simulink model "dram_acc_test8sim"  (Simulink 6.2)
settings: Solver=ode45  StartTime=0.0  StopTime=300000  RelTol=1e-3
undefined symbols (not defined in the file): ant_bits, blockCountBits, blockRowBits
libraries: xbsIndex_r3 x656, xps_library x19, casper_library x10
(part 4 of 4)

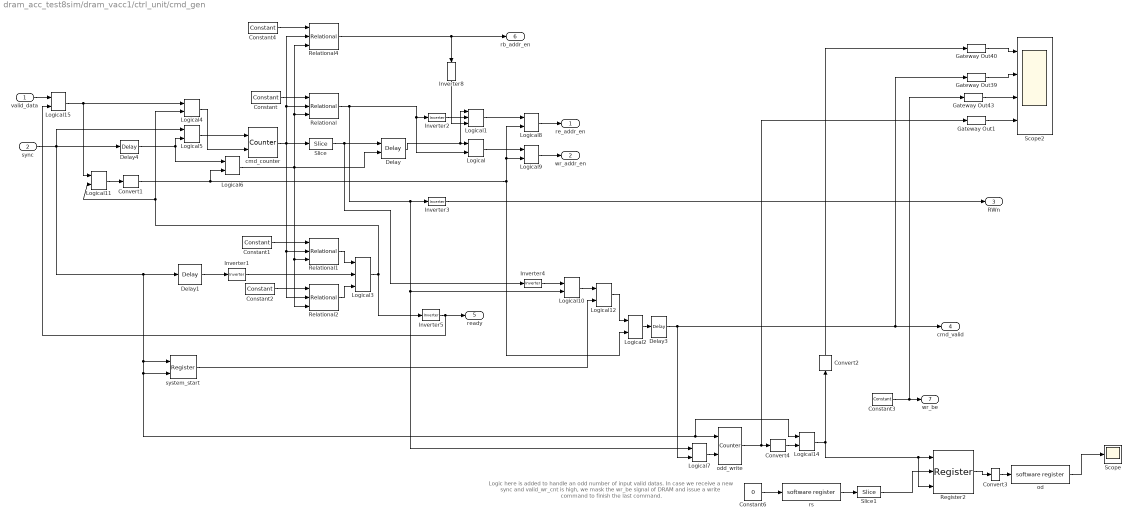
== system dram_acc_test8sim/dram_vacc1/ctrl_unit/cmd_gen ==
  note: Logic here is added to handle an  odd number of input valid datas.
      | In case we receive a new sync and valid_wr_cnt is high, we mask the wr_be
      | signal of DRAM and issue a write command to finish the last command.
  valid_data : Inport  Port=1  LatchInput=off
  sync : Inport  Port=2  LatchInput=off
  Constant : xbsIndex_r3/Constant  const=burst_length-1  equ=P=C  arith_type=Unsigned  n_bits=ceil(log2(2*burst_length+2))  bin_pt=0  opselect=C  inp2=PCIN>>17  opr=+  inp1=P  carry=CIN  iostate=0  explicit_period=on  period=1  dbl_ovrd=off
  Constant1 : xbsIndex_r3/Constant  const=burst_length-1  equ=P=C  arith_type=Unsigned  n_bits=ceil(log2(2*burst_length+2))  bin_pt=0  opselect=C  inp2=PCIN>>17  opr=+  inp1=P  carry=CIN  iostate=0  explicit_period=on  period=1  dbl_ovrd=off
  Constant2 : xbsIndex_r3/Constant  const=2*burst_length+2-1  equ=P=C  arith_type=Unsigned  n_bits=ceil(log2(2*burst_length+2))  bin_pt=0  opselect=C  inp2=PCIN>>17  opr=+  inp1=P  carry=CIN  iostate=0  explicit_period=on  period=1  dbl_ovrd=off
  Constant3 : xbsIndex_r3/Constant  const=2^18-1  equ=P=C  arith_type=Unsigned  n_bits=18  bin_pt=0  opselect=C  inp2=PCIN>>17  opr=+  inp1=P  carry=CIN  iostate=0  explicit_period=on  period=1  dbl_ovrd=off
  Constant4 : xbsIndex_r3/Constant  const=2*burst_length  equ=P=C  arith_type=Unsigned  n_bits=ceil(log2(2*burst_length+2))  bin_pt=0  opselect=C  inp2=PCIN>>17  opr=+  inp1=P  carry=CIN  iostate=0  explicit_period=on  period=1  dbl_ovrd=off
  Constant6 : Constant  Value=0
  Convert1 : xbsIndex_r3/Convert  arith_type=Boolean  n_bits=31  bin_pt=0  quantization=Truncate  overflow=Wrap  latency=0  explicit_period=on  period=1  dbl_ovrd=off  show_param=off  inserted_by_tool=off  pipeline=off
      settings: xl_area=[0, 0, 0, 0, 0, 0, 0]
  Convert2 : xbsIndex_r3/Convert  Orientation=up  arith_type=Boolean  n_bits=31  bin_pt=0  quantization=Truncate  overflow=Wrap  latency=1  explicit_period=on  period=1  dbl_ovrd=off  show_param=off  inserted_by_tool=off  pipeline=off
      settings: xl_area=[0, 0, 0, 0, 0, 0, 0]
  Convert3 : xbsIndex_r3/Convert  arith_type=Unsigned  n_bits=32  bin_pt=0  quantization=Truncate  overflow=Wrap  latency=0  explicit_period=on  period=1  dbl_ovrd=off  show_param=off  inserted_by_tool=off  pipeline=off
      settings: xl_area=[0, 0, 0, 0, 0, 0, 0]
  Convert4 : xbsIndex_r3/Convert  arith_type=Boolean  n_bits=31  bin_pt=0  quantization=Truncate  overflow=Wrap  latency=0  explicit_period=on  period=1  dbl_ovrd=off  show_param=off  inserted_by_tool=off  pipeline=off
      settings: xl_area=[0, 0, 0, 0, 0, 0, 0]
  Delay : xbsIndex_r3/Delay  latency=1  reg_retiming=off  explicit_period=off  period=1  en=on  accept_only_valid=off  init_zero=on  dbl_ovrd=off  show_param=off
      settings: xl_area=[0, 0, 0, 0, 0, 0, 0]
  Delay1 : xbsIndex_r3/Delay  latency=1  reg_retiming=off  explicit_period=off  period=1  en=off  accept_only_valid=off  init_zero=on  dbl_ovrd=off  show_param=off
      settings: xl_area=[0, 0, 0, 0, 0, 0, 0]
  Delay3 : xbsIndex_r3/Delay  latency=1  reg_retiming=off  explicit_period=on  period=1  en=off  accept_only_valid=off  init_zero=on  dbl_ovrd=off  show_param=off
      settings: xl_area=[0, 0, 0, 0, 0, 0, 0]
  Delay4 : xbsIndex_r3/Delay  latency=1  reg_retiming=off  explicit_period=on  period=1  en=off  accept_only_valid=off  init_zero=on  dbl_ovrd=off  show_param=off
      settings: xl_area=[0, 0, 0, 0, 0, 0, 0]
  Gateway Out{1,39..40,43} (4 alike) : xbsIndex_r3/Gateway Out  output_type=Double  nbits=8  bin_pt=6  arith_type=Boolean  quantization=Truncate  overflow=Wrap  hdl_port=off  timing_constraint=None  locs_specified=off  LOCs={}  needs_fixed_name=off  show_param=off
      settings: xl_area=[0, 0, 0, 0, 0, 0, 0]
  Inverter{1..5} (5 alike) : xbsIndex_r3/Inverter  latency=0  explicit_period=off  period=1  en=off  dbl_ovrd=off  show_param=off
      settings: xl_area=[0, 0, 0, 0, 0, 0, 0]
  Inverter8 : xbsIndex_r3/Inverter  Orientation=down  latency=0  explicit_period=off  period=1  en=off  dbl_ovrd=off  show_param=off
      settings: xl_area=[0, 0, 0, 0, 0, 0, 0]
  Logical{,2,7..9,12,14..15} (8 alike) : xbsIndex_r3/Logical  logical_function=AND  inputs=2  precision=Full  arith_type=Unsigned  n_bits=8  bin_pt=2  align_bp=on  latency=0  explicit_period=on  period=1  en=off  dbl_ovrd=off  show_param=off
      settings: xl_area=[0, 0, 0, 0, 0, 0, 0]
  Logical1 : xbsIndex_r3/Logical  logical_function=AND  inputs=3  precision=Full  arith_type=Unsigned  n_bits=8  bin_pt=2  align_bp=on  latency=0  explicit_period=on  period=1  en=off  dbl_ovrd=off  show_param=off
      settings: xl_area=[0, 0, 0, 0, 0, 0, 0]
  Logical10 : xbsIndex_r3/Logical  logical_function=OR  inputs=2  precision=Full  arith_type=Unsigned  n_bits=8  bin_pt=2  align_bp=on  latency=0  explicit_period=on  period=1  en=off  dbl_ovrd=off  show_param=off
      settings: xl_area=[0, 0, 0, 0, 0, 0, 0]
  Logical11 : xbsIndex_r3/Logical  logical_function=OR  inputs=2  precision=Full  arith_type=Unsigned  n_bits=8  bin_pt=2  align_bp=on  latency=0  explicit_period=on  period=1  en=off  dbl_ovrd=off  show_param=off
      settings: xl_area=[0, 0, 0, 0, 0, 0, 0]
  Logical3 : xbsIndex_r3/Logical  logical_function=AND  inputs=3  precision=Full  arith_type=Unsigned  n_bits=8  bin_pt=2  align_bp=on  latency=0  explicit_period=off  period=1  en=off  dbl_ovrd=off  show_param=off
      settings: xl_area=[0, 0, 0, 0, 0, 0, 0]
  Logical4 : xbsIndex_r3/Logical  logical_function=OR  inputs=2  precision=Full  arith_type=Unsigned  n_bits=8  bin_pt=2  align_bp=on  latency=0  explicit_period=off  period=1  en=off  dbl_ovrd=off  show_param=off
      settings: xl_area=[0, 0, 0, 0, 0, 0, 0]
  Logical5 : xbsIndex_r3/Logical  logical_function=OR  inputs=2  precision=Full  arith_type=Unsigned  n_bits=8  bin_pt=2  align_bp=on  latency=0  explicit_period=off  period=1  en=off  dbl_ovrd=off  show_param=off
      settings: xl_area=[0, 0, 0, 0, 0, 0, 0]
  Logical6 : xbsIndex_r3/Logical  logical_function=OR  inputs=2  precision=Full  arith_type=Unsigned  n_bits=8  bin_pt=2  align_bp=on  latency=0  explicit_period=on  period=1  en=off  dbl_ovrd=off  show_param=off
      settings: xl_area=[0, 0, 0, 0, 0, 0, 0]
  Register2 : xbsIndex_r3/Register  init=0  reg_only_valid=off  explicit_period=off  period=1  rst=on  en=on  out_en=off  dbl_ovrd=off  show_param=off
      settings: xl_area=[0, 0, 0, 0, 0, 0, 0]
  Relational : xbsIndex_r3/Relational  mode=a>=b  latency=1  explicit_period=on  period=1  en=on  dbl_ovrd=off  show_param=off
      settings: xl_area=[0, 0, 0, 0, 0, 0, 0]
  Relational1 : xbsIndex_r3/Relational  mode=a<=b  latency=1  explicit_period=on  period=1  en=on  dbl_ovrd=off  show_param=off
      settings: xl_area=[0, 0, 0, 0, 0, 0, 0]
  Relational2 : xbsIndex_r3/Relational  mode=a!=b  latency=1  explicit_period=off  period=1  en=on  dbl_ovrd=off  show_param=off
      settings: xl_area=[0, 0, 0, 0, 0, 0, 0]
  Relational4 : xbsIndex_r3/Relational  mode=a<=b  latency=1  explicit_period=on  period=1  en=on  dbl_ovrd=off  show_param=off
      settings: xl_area=[0, 0, 0, 0, 0, 0, 0]
  Scope : Scope
      settings: SaveName=ScopeData34
  Scope2 : Scope  NumInputPorts=4
      settings: YMin=-1~0~262143~0  YMax=1~1~262143~1  SaveName=ScopeData12
  Slice : xbsIndex_r3/Slice  mode=Lower Bit Location + Width  nbits=1  bit1=0  base1=MSB of Input  bit0=0  base0=LSB of Input  boolean_output=on  explicit_period=off  period=1  dbl_ovrd=off
  Slice1 : xbsIndex_r3/Slice  mode=Lower Bit Location + Width  nbits=1  bit1=0  base1=MSB of Input  bit0=0  base0=LSB of Input  boolean_output=on  explicit_period=off  period=1  dbl_ovrd=off
  cmd_counter : xbsIndex_r3/Counter  cnt_type=Count Limited  n_bits=ceil(log2(2*burst_length+2))  bin_pt=0  arith_type=Unsigned  start_count=0  cnt_to=2*burst_length+2-1  cnt_by_val=1  operation=Up  explicit_period=on  period=1  load_pin=off  rst=on  en=on  dbl_ovrd=off  show_param=off  use_rpm=on  gen_core=off
      settings: xl_area=[0, 0, 0, 0, 0, 0, 0]
  od : xps_library/software register  Tag=xps:sw_reg  io_dir=To Processor  arith_type=Unsigned  bitwidth=32  bin_pt=0  sample_period=1  gw_name=dram_acc_test8_dram_vacc1_ctrl_unit_cmd_gen_od_user_data_in
  odd_write : xbsIndex_r3/Counter  cnt_type=Free Running  n_bits=1  bin_pt=0  arith_type=Unsigned  start_count=0  cnt_to=2*burst_length+2-1  cnt_by_val=1  operation=Up  explicit_period=on  period=1  load_pin=off  rst=on  en=on  dbl_ovrd=off  show_param=off  use_rpm=on  gen_core=off
      settings: xl_area=[0, 0, 0, 0, 0, 0, 0]
  rs : xps_library/software register  Tag=xps:sw_reg  io_dir=From Processor  arith_type=Unsigned  bitwidth=32  bin_pt=0  sample_period=1  gw_name=dram_acc_test8_dram_vacc1_ctrl_unit_cmd_gen_rs_user_data_out
  system_start : xbsIndex_r3/Register  init=0  reg_only_valid=off  explicit_period=off  period=1  rst=off  en=on  out_en=off  dbl_ovrd=off  show_param=off
      settings: xl_area=[0, 0, 0, 0, 0, 0, 0]
  re_addr_en : Outport
  wr_addr_en : Outport  Port=2
  RWn : Outport  Port=3
  cmd_valid : Outport  Port=4
  ready : Outport  Port=5
  rb_addr_en : Outport  Port=6
  wr_be : Outport  Port=7
  wires:
  Logical9/1 -> wr_addr_en/1
  Logical8/1 -> re_addr_en/1
  Logical15/1 -> Logical4/1, Logical11/1
  Inverter8/1 -> Logical1/3
  Relational4/1 -> rb_addr_en/1, Inverter8/1
  Constant4/1 -> Relational4/1
  Logical6/1 -> Delay/2, Relational4/3, Relational/3, Relational1/3, Relational2/3
  Delay4/1 -> Logical6/1, Logical5/2
  Logical5/1 -> cmd_counter/1
  Logical2/1 -> Delay3/1
  Logical12/1 -> Logical2/1
  Convert1/1 -> Logical2/2, Logical8/2, Logical9/2, Logical6/2
  Inverter5/1 -> Logical15/2, ready/1
  Inverter4/1 -> Logical10/1
  Logical10/1 -> Logical12/1
  Inverter3/1 -> RWn/1
  Inverter2/1 -> Logical1/2
  system_start/1 -> Logical12/2
  Logical4/1 -> cmd_counter/2
  Logical3/1 -> Logical11/2, Logical4/2, Inverter5/1
  valid_data/1 -> Logical15/1
  Delay1/1 -> Inverter1/1
  Inverter1/1 -> Logical3/2
  Relational2/1 -> Logical3/3
  Constant2/1 -> Relational2/1
  Relational1/1 -> Logical3/1
  Constant1/1 -> Relational1/1
  Delay/1 -> Logical/1, Logical1/1
  Relational/1 -> Inverter3/1, Logical10/2, Logical7/1, Logical/2, Inverter2/1
  Slice/1 -> Inverter4/1, Delay/1
  Logical1/1 -> Logical8/1
  Logical/1 -> Logical9/1
  Logical11/1 -> Convert1/1
  Constant/1 -> Relational/1
  cmd_counter/1 -> Relational2/2, Relational1/2, Relational4/2, Relational/2, Slice/1
  sync/1 -> Delay4/1, Logical5/1, system_start/1, system_start/2, odd_write/1, Logical14/1, Delay1/1
  Logical7/1 -> odd_write/2
  odd_write/1 -> Convert4/1, Gateway Out1/1
  Logical14/1 -> Register2/1, Register2/3, Convert2/1
  Constant3/1 -> wr_be/1, Gateway Out43/1
  Delay3/1 -> Logical7/2, cmd_valid/1, Gateway Out39/1
  Convert2/1 -> Gateway Out40/1
  Convert4/1 -> Logical14/2
  Gateway Out43/1 -> Scope2/3
  Gateway Out39/1 -> Scope2/2
  Gateway Out40/1 -> Scope2/1
  Gateway Out1/1 -> Scope2/4
  rs/1 -> Slice1/1
  Slice1/1 -> Register2/2
  Constant6/1 -> rs/1
  Register2/1 -> Convert3/1
  od/1 -> Scope/1
  Convert3/1 -> od/1

== system dram_acc_test8sim/dram_vacc1/ctrl_unit/latch_rb_enable ==
  sync : Inport  Port=1  LatchInput=off
  rb_addr_enable : Inport  Port=2  LatchInput=off
  negedge : Inport  Port=3  LatchInput=off
  Inverter5 : xbsIndex_r3/Inverter  latency=0  explicit_period=off  period=1  en=off  dbl_ovrd=off  show_param=off
      settings: xl_area=[0, 0, 0, 0, 0, 0, 0]
  Logical1 : xbsIndex_r3/Logical  logical_function=OR  inputs=2  precision=Full  arith_type=Unsigned  n_bits=8  bin_pt=2  align_bp=on  latency=0  explicit_period=on  period=1  en=off  dbl_ovrd=off  show_param=off
      settings: xl_area=[0, 0, 0, 0, 0, 0, 0]
  Logical2 : xbsIndex_r3/Logical  logical_function=OR  inputs=2  precision=Full  arith_type=Unsigned  n_bits=8  bin_pt=2  align_bp=on  latency=1  explicit_period=on  period=1  en=off  dbl_ovrd=off  show_param=off
      settings: xl_area=[0, 0, 0, 0, 0, 0, 0]
  Logical3 : xbsIndex_r3/Logical  logical_function=AND  inputs=2  precision=Full  arith_type=Unsigned  n_bits=8  bin_pt=2  align_bp=on  latency=0  explicit_period=on  period=1  en=off  dbl_ovrd=off  show_param=off
      settings: xl_area=[0, 0, 0, 0, 0, 0, 0]
  Logical4 : xbsIndex_r3/Logical  logical_function=AND  inputs=2  precision=Full  arith_type=Unsigned  n_bits=8  bin_pt=2  align_bp=on  latency=0  explicit_period=on  period=1  en=off  dbl_ovrd=off  show_param=off
      settings: xl_area=[0, 0, 0, 0, 0, 0, 0]
  system_start3 : xbsIndex_r3/Register  init=0  reg_only_valid=off  explicit_period=off  period=1  rst=off  en=on  out_en=off  dbl_ovrd=off  show_param=off
      settings: xl_area=[0, 0, 0, 0, 0, 0, 0]
  inc_addr_en : Outport
  cmd_tag : Outport  Port=2
  wires:
  Inverter5/1 -> Logical4/2
  Logical3/1 -> inc_addr_en/1
  negedge/1 -> system_start3/2, Logical3/2, Inverter5/1
  rb_addr_enable/1 -> Logical1/2
  sync/1 -> Logical1/1
  Logical4/1 -> Logical2/1
  Logical2/1 -> Logical4/1, system_start3/1
  Logical1/1 -> Logical2/2
  system_start3/1 -> cmd_tag/1, Logical3/1

== system dram_acc_test8sim/dram_vacc1/ctrl_unit/negedge ==
  in : Inport  Port=1  LatchInput=off
  Delay : xbsIndex_r3/Delay  latency=1  reg_retiming=off  explicit_period=off  period=1  en=off  accept_only_valid=off  init_zero=on  dbl_ovrd=off  show_param=off
      settings: xl_area=[0, 0, 0, 0, 0, 0, 0]
  Inverter1 : xbsIndex_r3/Inverter  latency=0  explicit_period=off  period=1  en=off  dbl_ovrd=off  show_param=off
      settings: xl_area=[0, 0, 0, 0, 0, 0, 0]
  Logical : xbsIndex_r3/Logical  logical_function=AND  inputs=2  precision=Full  arith_type=Unsigned  n_bits=8  bin_pt=2  align_bp=on  latency=0  explicit_period=off  period=1  en=off  dbl_ovrd=off  show_param=off
      settings: xl_area=[0, 0, 0, 0, 0, 0, 0]
  out : Outport
  wires:
  Inverter1/1 -> Logical/2
  Delay/1 -> Logical/1
  in/1 -> Inverter1/1, Delay/1
  Logical/1 -> out/1

== system dram_acc_test8sim/dram_vacc1/ctrl_unit/readback_address_dram_vacc ==
  sync : Inport  Port=1  LatchInput=off
  en : Inport  Port=2  LatchInput=off
  block_counter : xbsIndex_r3/Counter  cnt_type=Free Running  n_bits=blockCountBits  bin_pt=0  arith_type=Unsigned  start_count=2^blockCountBits-2  cnt_to=Inf  cnt_by_val=1  operation=Up  explicit_period=off  period=1  load_pin=off  rst=off  en=on  dbl_ovrd=off  show_param=off  use_rpm=on  gen_core=off
      settings: xl_area=[0, 0, 0, 0, 0, 0, 0]
  cast1 : xbsIndex_r3/Convert  arith_type=Unsigned  n_bits=8  bin_pt=0  quantization=Truncate  overflow=Wrap  latency=0  explicit_period=off  period=1  dbl_ovrd=off  show_param=off  inserted_by_tool=off  pipeline=off
      settings: xl_area=[0, 0, 0, 0, 0, 0, 0]
  concat1 : xbsIndex_r3/Concat  num_inputs=2  explicit_period=off  period=1  dbl_ovrd=off
  concat3 : xbsIndex_r3/Concat  num_inputs=6  explicit_period=off  period=1  dbl_ovrd=off
  const0 : xbsIndex_r3/Constant  const=0  equ=P=C  arith_type=Unsigned  n_bits=5  bin_pt=0  opselect=C  inp2=PCIN>>17  opr=+  inp1=P  carry=CIN  iostate=0  explicit_period=off  period=1  dbl_ovrd=off
  const1 : xbsIndex_r3/Constant  const=0  equ=P=C  arith_type=Unsigned  n_bits=2  bin_pt=0  opselect=C  inp2=PCIN>>17  opr=+  inp1=P  carry=CIN  iostate=0  explicit_period=off  period=1  dbl_ovrd=off
  read_counter : xbsIndex_r3/Counter  cnt_type=Count Limited  n_bits=counterBitWidth  bin_pt=0  arith_type=Unsigned  start_count=0  cnt_to=acc_length/2-1  cnt_by_val=1  operation=Up  explicit_period=off  period=1  load_pin=on  rst=on  en=on  dbl_ovrd=off  show_param=off  use_rpm=on  gen_core=off
      settings: xl_area=[0, 0, 0, 0, 0, 0, 0]
  slice10 : xbsIndex_r3/Slice  mode=Lower Bit Location + Width  nbits=2  bit1=0  base1=MSB of Input  bit0=0  base0=LSB of Input  boolean_output=off  explicit_period=off  period=1  dbl_ovrd=off
  slice11 : xbsIndex_r3/Slice  mode=Upper Bit Location + Width  nbits=blockCountBits-2  bit1=0  base1=MSB of Input  bit0=0  base0=LSB of Input  boolean_output=off  explicit_period=off  period=1  dbl_ovrd=off
  slice14 : xbsIndex_r3/Slice  mode=Upper Bit Location + Width  nbits=1  bit1=0  base1=MSB of Input  bit0=0  base0=LSB of Input  boolean_output=off  explicit_period=off  period=1  dbl_ovrd=off
  slice15 : xbsIndex_r3/Slice  mode=Lower Bit Location + Width  nbits=blockCountBits-3  bit1=0  base1=MSB of Input  bit0=0  base0=LSB of Input  boolean_output=off  explicit_period=off  period=1  dbl_ovrd=off
  slice6 : xbsIndex_r3/Slice  mode=Lower Bit Location + Width  nbits=colCountBits  bit1=0  base1=MSB of Input  bit0=0  base0=LSB of Input  boolean_output=off  explicit_period=off  period=1  dbl_ovrd=off
  slice7 : xbsIndex_r3/Slice  mode=Upper Bit Location + Width  nbits=blockCountBits+blockRowBits  bit1=0  base1=MSB of Input  bit0=0  base0=LSB of Input  boolean_output=off  explicit_period=off  period=1  dbl_ovrd=off
  slice9 : xbsIndex_r3/Slice  mode=Upper Bit Location + Width  nbits=blockCountBits  bit1=0  base1=MSB of Input  bit0=0  base0=LSB of Input  boolean_output=off  explicit_period=off  period=1  dbl_ovrd=off
  readback_addr : Outport
  wires:
  const1/1 -> concat3/1
  slice10/1 -> concat3/2
  slice15/1 -> concat3/3
  slice14/1 -> concat3/4
  cast1/1 -> concat3/5
  const0/1 -> concat3/6
  sync/1 -> read_counter/1, block_counter/1
  en/1 -> read_counter/2
  block_counter/1 -> concat1/1
  read_counter/1 -> concat1/2
  concat1/1 -> slice6/1, slice7/1
  slice6/1 -> cast1/1
  slice7/1 -> slice9/1
  slice9/1 -> slice10/1, slice11/1
  concat3/1 -> readback_addr/1
  slice11/1 -> slice14/1, slice15/1

== system dram_acc_test8sim/dram_vacc1/dram1/sim_wrapper ==
  rst : Inport  Port=1  LatchInput=off
  address : Inport  Port=2  LatchInput=off
  data_in : Inport  Port=3  LatchInput=off
  wr_be : Inport  Port=4  LatchInput=off
  RWn : Inport  Port=5  LatchInput=off
  cmd_tag : Inport  Port=6  LatchInput=off
  cmd_valid : Inport  Port=7  LatchInput=off
  rd_ack : Inport  Port=8  LatchInput=off
  Disregard Subsystem : xbsIndex_r3/Disregard Subsystem  Tag=discardX
      settings: AttributesFormatString=Disregard Subsystem\nFor Generation
  ModelSim : xbsIndex_r3/ModelSim  dir=./modelsim  waveform=on  leave_open=on  skip_compile=off  custom_scripts=off  post_vsim_script=dram_sim.do  startup_timeout=600
  Terminator : Terminator
  Terminator1 : Terminator
  dram_sim : xbsIndex_r3/Black Box  init_code=dram_sim  sim_method=Use HDL Co-Simulation  engine_block=../../../ModelSim  show_param=off
      settings: xl_area=[0, 0, 0, 0, 0, 0, 0]
  cmd_ack : Outport
  data_out : Outport  Port=2
  rd_tag : Outport  Port=3
  rd_valid : Outport  Port=4
  wires:
  rst/1 -> dram_sim/1
  dram_sim/1 -> cmd_ack/1
  dram_sim/2 -> data_out/1
  dram_sim/3 -> rd_tag/1
  dram_sim/4 -> rd_valid/1
  dram_sim/5 -> Terminator/1
  dram_sim/6 -> Terminator1/1
  address/1 -> dram_sim/2
  data_in/1 -> dram_sim/3
  wr_be/1 -> dram_sim/4
  RWn/1 -> dram_sim/5
  cmd_tag/1 -> dram_sim/6
  cmd_valid/1 -> dram_sim/7
  rd_ack/1 -> dram_sim/8

== system dram_acc_test8sim/dram_vacc1/fifo_empty_check/negedge ==
  in : Inport  Port=1  LatchInput=off
  Delay : xbsIndex_r3/Delay  latency=1  reg_retiming=off  explicit_period=off  period=1  en=off  accept_only_valid=off  init_zero=on  dbl_ovrd=off  show_param=off
      settings: xl_area=[0, 0, 0, 0, 0, 0, 0]
  Inverter1 : xbsIndex_r3/Inverter  latency=0  explicit_period=off  period=1  en=off  dbl_ovrd=off  show_param=off
      settings: xl_area=[0, 0, 0, 0, 0, 0, 0]
  Logical : xbsIndex_r3/Logical  logical_function=AND  inputs=2  precision=Full  arith_type=Unsigned  n_bits=8  bin_pt=2  align_bp=on  latency=0  explicit_period=off  period=1  en=off  dbl_ovrd=off  show_param=off
      settings: xl_area=[0, 0, 0, 0, 0, 0, 0]
  out : Outport
  wires:
  Inverter1/1 -> Logical/2
  Logical/1 -> out/1
  in/1 -> Inverter1/1, Delay/1
  Delay/1 -> Logical/1

== system dram_acc_test8sim/dram_vacc1/Adder/initializer/posedge ==
  in : Inport  Port=1  LatchInput=off
  Delay : xbsIndex_r3/Delay  latency=1  reg_retiming=off  explicit_period=off  period=1  en=off  accept_only_valid=off  init_zero=on  dbl_ovrd=off  show_param=off
      settings: xl_area=[0, 0, 0, 0, 0, 0, 0]
  Inverter2 : xbsIndex_r3/Inverter  latency=0  explicit_period=off  period=1  en=off  dbl_ovrd=off  show_param=off
      settings: xl_area=[0, 0, 0, 0, 0, 0, 0]
  Logical : xbsIndex_r3/Logical  logical_function=AND  inputs=2  precision=Full  arith_type=Unsigned  n_bits=8  bin_pt=2  align_bp=on  latency=0  explicit_period=off  period=1  en=off  dbl_ovrd=off  show_param=off
      settings: xl_area=[0, 0, 0, 0, 0, 0, 0]
  out : Outport
  wires:
  Inverter2/1 -> Logical/1
  Logical/1 -> out/1
  in/1 -> Logical/2, Delay/1
  Delay/1 -> Inverter2/1

== system dram_acc_test8sim/dram_vacc1/Adder/initializer/posedge1 ==
  in : Inport  Port=1  LatchInput=off
  Delay : xbsIndex_r3/Delay  latency=1  reg_retiming=off  explicit_period=off  period=1  en=off  accept_only_valid=off  init_zero=on  dbl_ovrd=off  show_param=off
      settings: xl_area=[0, 0, 0, 0, 0, 0, 0]
  Inverter2 : xbsIndex_r3/Inverter  latency=0  explicit_period=off  period=1  en=off  dbl_ovrd=off  show_param=off
      settings: xl_area=[0, 0, 0, 0, 0, 0, 0]
  Logical : xbsIndex_r3/Logical  logical_function=AND  inputs=2  precision=Full  arith_type=Unsigned  n_bits=8  bin_pt=2  align_bp=on  latency=0  explicit_period=off  period=1  en=off  dbl_ovrd=off  show_param=off
      settings: xl_area=[0, 0, 0, 0, 0, 0, 0]
  out : Outport
  wires:
  Delay/1 -> Inverter2/1
  in/1 -> Delay/1, Logical/2
  Logical/1 -> out/1
  Inverter2/1 -> Logical/1

== system dram_acc_test8sim/dram_vacc1/Adder/initializer/posedge2 ==
  in : Inport  Port=1  LatchInput=off
  Delay : xbsIndex_r3/Delay  latency=1  reg_retiming=off  explicit_period=off  period=1  en=off  accept_only_valid=off  init_zero=on  dbl_ovrd=off  show_param=off
      settings: xl_area=[0, 0, 0, 0, 0, 0, 0]
  Inverter2 : xbsIndex_r3/Inverter  latency=0  explicit_period=off  period=1  en=off  dbl_ovrd=off  show_param=off
      settings: xl_area=[0, 0, 0, 0, 0, 0, 0]
  Logical : xbsIndex_r3/Logical  logical_function=AND  inputs=2  precision=Full  arith_type=Unsigned  n_bits=8  bin_pt=2  align_bp=on  latency=0  explicit_period=off  period=1  en=off  dbl_ovrd=off  show_param=off
      settings: xl_area=[0, 0, 0, 0, 0, 0, 0]
  out : Outport
  wires:
  Inverter2/1 -> Logical/1
  Logical/1 -> out/1
  in/1 -> Logical/2, Delay/1
  Delay/1 -> Inverter2/1

== system dram_acc_test8sim/dram_vacc1/Adder/initializer/posedge3 ==
  in : Inport  Port=1  LatchInput=off
  Delay : xbsIndex_r3/Delay  latency=1  reg_retiming=off  explicit_period=off  period=1  en=off  accept_only_valid=off  init_zero=on  dbl_ovrd=off  show_param=off
      settings: xl_area=[0, 0, 0, 0, 0, 0, 0]
  Inverter2 : xbsIndex_r3/Inverter  latency=0  explicit_period=off  period=1  en=off  dbl_ovrd=off  show_param=off
      settings: xl_area=[0, 0, 0, 0, 0, 0, 0]
  Logical : xbsIndex_r3/Logical  logical_function=AND  inputs=2  precision=Full  arith_type=Unsigned  n_bits=8  bin_pt=2  align_bp=on  latency=0  explicit_period=off  period=1  en=off  dbl_ovrd=off  show_param=off
      settings: xl_area=[0, 0, 0, 0, 0, 0, 0]
  out : Outport
  wires:
  Delay/1 -> Inverter2/1
  in/1 -> Delay/1, Logical/2
  Logical/1 -> out/1
  Inverter2/1 -> Logical/1

== system dram_acc_test8sim/dram_vacc1/Adder/initializer/posedge4 ==
  in : Inport  Port=1  LatchInput=off
  Delay : xbsIndex_r3/Delay  latency=1  reg_retiming=off  explicit_period=off  period=1  en=off  accept_only_valid=off  init_zero=on  dbl_ovrd=off  show_param=off
      settings: xl_area=[0, 0, 0, 0, 0, 0, 0]
  Inverter2 : xbsIndex_r3/Inverter  latency=0  explicit_period=off  period=1  en=off  dbl_ovrd=off  show_param=off
      settings: xl_area=[0, 0, 0, 0, 0, 0, 0]
  Logical : xbsIndex_r3/Logical  logical_function=AND  inputs=2  precision=Full  arith_type=Unsigned  n_bits=8  bin_pt=2  align_bp=on  latency=0  explicit_period=off  period=1  en=off  dbl_ovrd=off  show_param=off
      settings: xl_area=[0, 0, 0, 0, 0, 0, 0]
  out : Outport
  wires:
  Inverter2/1 -> Logical/1
  Logical/1 -> out/1
  in/1 -> Logical/2, Delay/1
  Delay/1 -> Inverter2/1

== system dram_acc_test8sim/dram_vacc1/Adder/initializer/posedge5 ==
  in : Inport  Port=1  LatchInput=off
  Delay : xbsIndex_r3/Delay  latency=1  reg_retiming=off  explicit_period=off  period=1  en=off  accept_only_valid=off  init_zero=on  dbl_ovrd=off  show_param=off
      settings: xl_area=[0, 0, 0, 0, 0, 0, 0]
  Inverter2 : xbsIndex_r3/Inverter  latency=0  explicit_period=off  period=1  en=off  dbl_ovrd=off  show_param=off
      settings: xl_area=[0, 0, 0, 0, 0, 0, 0]
  Logical : xbsIndex_r3/Logical  logical_function=AND  inputs=2  precision=Full  arith_type=Unsigned  n_bits=8  bin_pt=2  align_bp=on  latency=0  explicit_period=off  period=1  en=off  dbl_ovrd=off  show_param=off
      settings: xl_area=[0, 0, 0, 0, 0, 0, 0]
  out : Outport
  wires:
  Delay/1 -> Inverter2/1
  in/1 -> Delay/1, Logical/2
  Logical/1 -> out/1
  Inverter2/1 -> Logical/1
